simulink subsystem "FR_Load_Diff"  (R2021b)
settings: Solver=VariableStepAuto  StartTime=0.0  StopTime=10.0  RelTol=1e-3
undefined symbols (not defined in the file): cf, g, hg, kf, kt, l, M, m1f, m2f, W0_F, W0_R
settings Model: Creator=tsuyoshi  LastModifiedBy=tsuyoshi

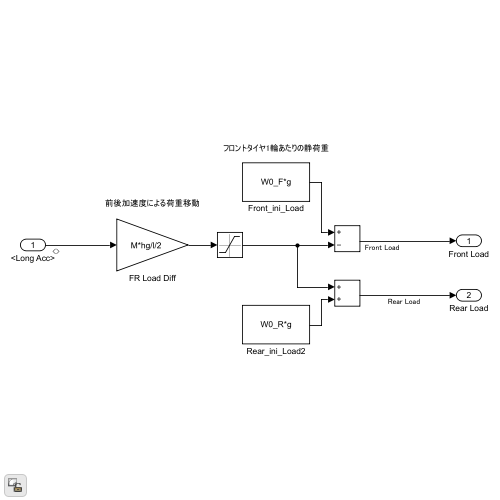
[thumbnail: Simulink's stored preview of the top-level diagram]
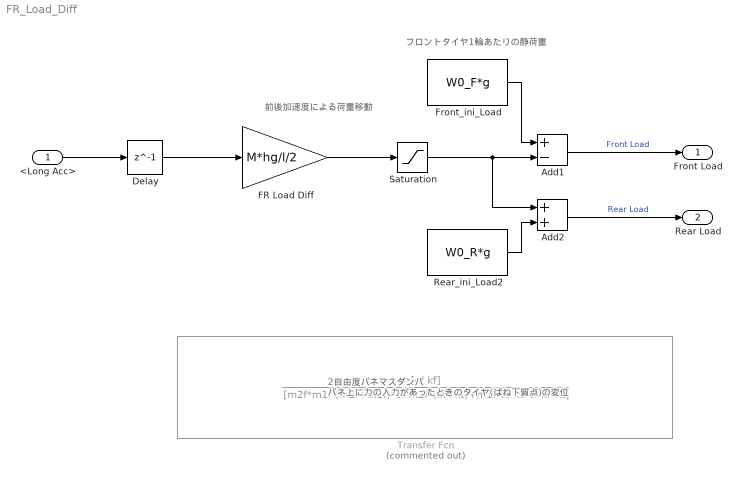
== system FR_Load_Diff ==
  note: 2自由度バネマスダンパ
      | バネ上に力の入力があったときのタイヤ(ばね下質点)の変位
  note: 前後加速度による荷重移動
  note: フロントタイヤ1輪あたりの静荷重
  <Long Acc> : Inport
  Add1 : Sum  Inputs=+-
  Add2 : Sum
  Delay : Delay  DelayLength=1
  FR Load Diff : Gain  Gain=M*hg/l/2
  Front_ini_Load : Constant  Value=W0_F*g
  Rear_ini_Load2 : Constant  Value=W0_R*g
  Saturation : Saturate  UpperLimit=W0_F*9.8  LowerLimit=W0_R*(-9.8)
  Transfer Fcn : TransferFcn  Commented=on  Numerator=[cf kf]  Denominator=[m2f*m1f (m2f+m1f)*cf m2f*(kf+kt)+m1f*kf kt*cf kf*kt]
  Front Load : Outport
  Rear Load : Outport  Port=2
  wires:
  Rear_ini_Load2/1 -> Add2/2
  FR Load Diff/1 -> Saturation/1
  Add2/1 -> Rear Load/1  "Rear Load"
  Saturation/1 -> Add1/2, Add2/1
  Front_ini_Load/1 -> Add1/1
  <Long Acc>/1 -> Delay/1
  Add1/1 -> Front Load/1  "Front Load"
  Delay/1 -> FR Load Diff/1
